simulink model "MotorModelVariableSeparateRotors"  (R2015b)
settings: Solver=VariableStepAuto  StartTime=0.0  StopTime=10.0  RelTol=1e-3
undefined symbols (not defined in the file): Initial, Motor, Uav
settings Model: Creator=jban039  LastModifiedBy=jban039

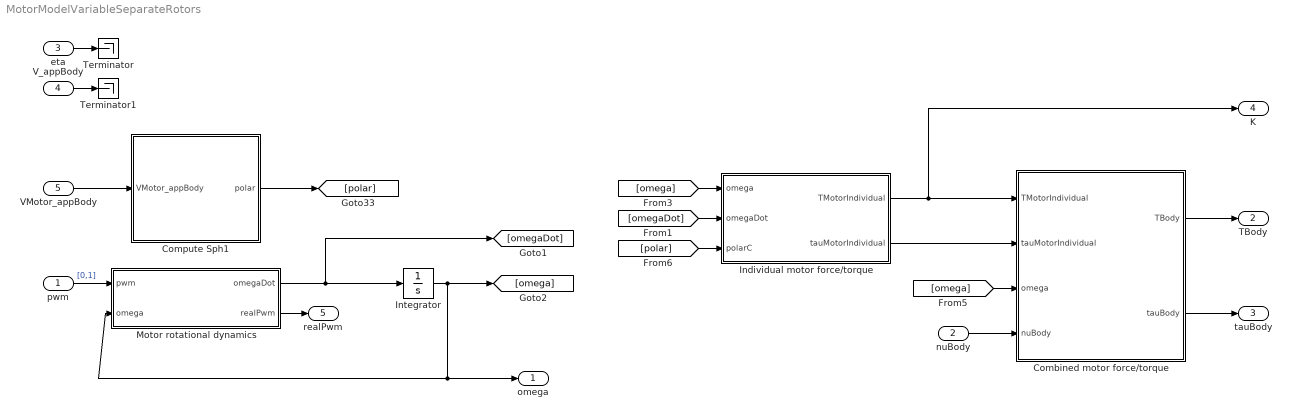
== system MotorModelVariableSeparateRotors ==
  pwm : Inport  PortDimensions=Uav.N_ROTORS
  nuBody : Inport  Port=2  PortDimensions=3
  eta : Inport  Port=3  PortDimensions=3
  V_appBody : Inport  Port=4  PortDimensions=3
  VMotor_appBody : Inport  Port=5  PortDimensions=[3,4]
  Combined motor force/torque : MATLAB Function  TreatAsAtomicUnit=on
  Compute Sph1 : MATLAB Function  TreatAsAtomicUnit=on
  Individual motor force/torque : MATLAB Function  TreatAsAtomicUnit=on
  Integrator : Integrator  InitialCondition=Initial.OMEGA
  Motor rotational dynamics : MATLAB Function  TreatAsAtomicUnit=on
  Terminator : Terminator
  Terminator1 : Terminator
  omega : Outport
  TBody : Outport  Port=2
  tauBody : Outport  Port=3
  K : Outport  Port=4
  realPwm : Outport  Port=5
  wires:
  Combined motor force/torque/2(tauBody) -> tauBody/1
  Combined motor force/torque/1(TBody) -> TBody/1
  pwm/1 -> Motor rotational dynamics/1(pwm)  "[0,1]"
  eta/1 -> Terminator/1
  Individual motor force/torque/2(tauMotorIndividual) -> Combined motor force/torque/2(tauMotorIndividual)
  Motor rotational dynamics/1(omegaDot) -> [omegaDot], Integrator/1
  nuBody/1 -> Combined motor force/torque/4(nuBody)
  Compute Sph1/1(polar) -> [polar]
  Individual motor force/torque/1(TMotorIndividual) -> Combined motor force/torque/1(TMotorIndividual), K/1
  [omegaDot] -> Individual motor force/torque/2(omegaDot)
  Integrator/1 -> [omega], Motor rotational dynamics/2(omega), omega/1
  [omega] -> Individual motor force/torque/1(omega)
  [omega] -> Combined motor force/torque/3(omega)
  [polar] -> Individual motor force/torque/3(polarC)
  Motor rotational dynamics/2(realPwm) -> realPwm/1
  VMotor_appBody/1 -> Compute Sph1/1(VMotor_appBody)
  V_appBody/1 -> Terminator1/1

== matlab function MotorModelVariableSeparateRotors/Compute Sph1 ==
  data: VMotor_appBody input; polar output
function polar  = computeSph(VMotor_appBody)
%#codegen

% Convert from polar to spherical coordinates
radius = zeros(1,4);
elevation = zeros(1,4);
azimuth = zeros(1,4);

for i = 1:length( radius )
    [ azimuth(1,i), elevation(1,i), radius(1,i) ] = ...
        cart2sph( VMotor_appBody(1,i), VMotor_appBody(2,i), VMotor_appBody(3,i) );
end


polar = [azimuth; elevation; radius];

== matlab function MotorModelVariableSeparateRotors/Individual motor force//torque ==
  data: omega input; TMotorIndividual output size=[3 4]; omegaDot input; polarC input; Motor parameter; Uav parameter; tauMotorIndividual output size=[3 4]
function [TMotorIndividual, tauMotorIndividual] = motorIndividual( ...
    omega, omegaDot, polarC, Motor, Uav)
%#codegen

elevation = polarC(2,:);
windSpeed = polarC(3,:);

% Make assertions to avoid code generation errors
assert(Uav.N_ROTORS < 16);

%% Thrust and differential torque

% Concatenated motor force/torque vectors in respective motor frame
% eg. TMotor = [TMotor1, TMotor2, ..., TMotorN]
% where: - N is the number of rotors
%        - TMotorx (x ∈ [1,2,...,N]) is the thrust generated by motor x in
%          its own frame of reference
% TMotorIndividual = [ zeros(2, Uav.N_ROTORS);
%                      K * (omega'.^2) ];

K1 = 6.543988868292138e-05 + ...
     1.886359198743874e-06 * sin(-elevation) + ...
    -7.693938774360465e-07 * windSpeed + ...
     2.639630950517221e-06 * sin(-elevation) .* windSpeed + ...
     2.126334444415667e-08 * windSpeed.^2;
K2 = -1.903771811601254e-04 + ...
      2.812570127999989e-03 * sin(-elevation) + ...
      1.418616236881443e-03 * windSpeed + ...
     -4.525882966383329e-03 * sin(-elevation) .* windSpeed + ...
     -1.658875316836167e-05 * windSpeed.^2;
 
 % RECOMPUTE THRUST COEFFICIENTS AS CURRENT VALUES OUT BY FACTOR OF 4

TMotorIndividual = [ zeros(2, Uav.N_ROTORS);
                     0.25 * 0.5 * Uav.RHO_AIR * K1 .* (omega'.^2) + ...
                     0.25 * 0.5 * Uav.RHO_AIR * K2 .* (omega') ];

tauMotorIndividual = [ zeros(2, Uav.N_ROTORS);
                      -Uav.ROTOR_DIRECTION .* ...
                      ( Motor.B * (omega'.^2) + Motor.I_R(3,3) * omegaDot' ) ];

== matlab function MotorModelVariableSeparateRotors/Motor rotational dynamics ==
  data: pwm input; omegaDot output; omega input; realPwm output
function [omegaDot, realPwm]  = motorRotDynamics( pwm, omega)
%#codegen

realPwm = (1000 * pwm + 1000);
realPwm(2) = realPwm(2) - 200;
realPwm(4) = realPwm(4) - 200;

realPwm( realPwm < 1230 ) = 1230;

rotorTimeConst = 7.006512e-02;
omegaRef = 7.969173e-1 * realPwm - 6.528579e2;
omegaDot = (omegaRef - omega) / rotorTimeConst;

== matlab function MotorModelVariableSeparateRotors/Combined motor force//torque ==
  data: TMotorIndividual input; TBody output size=3; tauMotorIndividual input; tauBody output size=3; omega input; nuBody input; Motor parameter; Uav parameter
function [TBody, tauBody] = motorCombined( TMotorIndividual,tauMotorIndividual,  ...
    omega, nuBody, Motor, Uav)
%#codegen
assert(Uav.N_ROTORS < 16);

% Initialise matrices to store motor force/torque vectors in body frame
TBodyIndividual   = zeros(3, Uav.N_ROTORS);
tauBodyIndividual = zeros(3, Uav.N_ROTORS);

% Calculate forces and moments from each motor in the body frame
for i = 1:Uav.N_ROTORS
    l = Uav.L(i);
    beta = Uav.BETA(i);
    
    % Matrix to compute torque applied by rotor thrust
 	L = [ 0,            0,            l*sin(beta);
          0,            0,           -l*cos(beta);
         -l*sin(beta),  l*cos(beta),  0 ];

	% Motor force/torque vectors in body frame
	TBodyIndividual(:,i) = Uav.R_MOTOR_TO_BODY(:,:,i) * ...
        TMotorIndividual(:,i);
	tauBodyIndividual(:,i) = Uav.R_MOTOR_TO_BODY(:,:,i) * ...
        tauMotorIndividual(:,i) + L * TBodyIndividual(:,i);
end

%% Gyroscopic moments

% Concatenated gyroscopic moments for each rotor
M_GBodyIndividual = zeros(3, Uav.N_ROTORS);

% Concatenated motor speeds in their respective frames
omegaMotor = [ zeros(2, Uav.N_ROTORS);
               Uav.ROTOR_DIRECTION .* omega' ];

% Angular momentum in motor frame
H_MMotorSeparate = Motor.I_R * omegaMotor;

% Gyroscopic moment vectors in body frame
for i = 1:Uav.N_ROTORS
	M_GBodyIndividual(:,i) = cross( nuBody, ...
        Uav.R_MOTOR_TO_BODY(:,:,i) * H_MMotorSeparate(:,i) );
end

M_GBody = sum(M_GBodyIndividual, 2);

%% Total torque and moment

% Total force/torque in body frame
TBody = sum(TBodyIndividual, 2);
tauBody = sum(tauBodyIndividual, 2) - M_GBody;

end
